simulink model "Potenciometro"  (R2022b)
settings: Solver=VariableStepAuto  StartTime=0.0  StopTime=10.0  RelTol=1e-3
libraries: fl_lib x6, nesl_utility x2, ee_lib x1
settings Model: Creator=matheusassis  LastModifiedBy=matheusassis

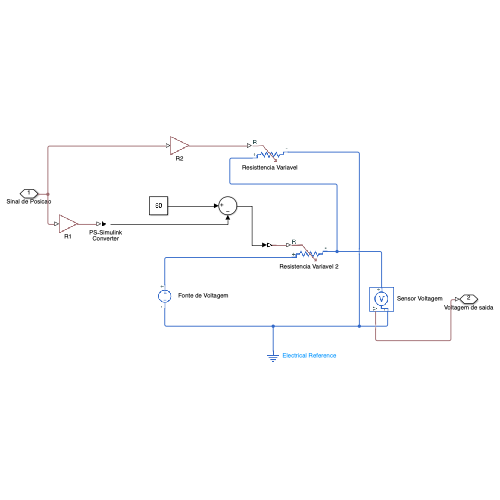
[thumbnail: Simulink's stored preview of the top-level diagram]
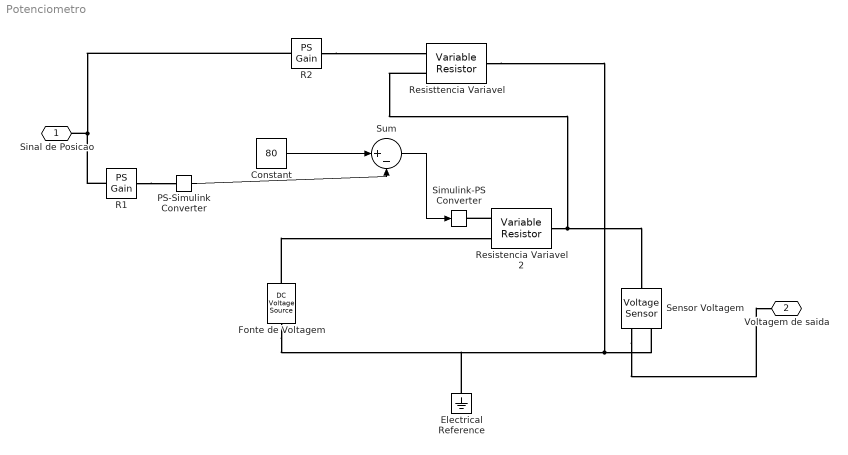
== system Potenciometro ==
  " Fonte de Voltagem" : ee_lib/Additional Components/SPICE Sources/DC Voltage Source  DC=10 V
  Constant : Constant  Value=80
  Electrical Reference : fl_lib/Electrical/Electrical Elements/Electrical Reference
  PS-Simulink Converter : nesl_utility/PS-Simulink Converter  PhysicalDomain=network_engine_domain  SubClassName=ps_output  LeftPortType=input  RightPortType=output  PseudoPeriodic=off  Frequencies=[]  VectorFormat=inherit  Unit=inherit  AffineConversion=off
  R1 : fl_lib/Physical Signals/Functions/PS Gain  gain=1
  R2 : fl_lib/Physical Signals/Functions/PS Gain  gain=1
  Resistencia Variavel 2 : fl_lib/Electrical/Electrical Elements/Variable Resistor  Rmin=0 Ohm  i_specify=off  i_priority=None  i=0 A  i_nominal_specify=off  i_nominal_unit=A  i_nominal_value=1  v_specify=off  v_priority=None  v=0 V  v_nominal_specify=off  v_nominal_unit=V  v_nominal_value=1
  Resisttencia Variavel : fl_lib/Electrical/Electrical Elements/Variable Resistor  Rmin=0 Ohm  i_specify=off  i_priority=None  i=0 A  i_nominal_specify=off  i_nominal_unit=A  i_nominal_value=1  v_specify=off  v_priority=None  v=0 V  v_nominal_specify=off  v_nominal_unit=V  v_nominal_value=1
  "Sensor Voltagem " : fl_lib/Electrical/Electrical Sensors/Voltage Sensor
  Simulink-PS Converter : nesl_utility/Simulink-PS Converter  PhysicalDomain=network_engine_domain  SubClassName=ps_input  LeftPortType=input  RightPortType=output  PseudoPeriodic=off  Frequencies=[]  NoiseDistribution=none  NoiseParameters=[]  Unit=1  AffineConversion=off  FilteringAndDerivatives=provide  SimscapeFilterOrder=1  InputFilterTimeConstant=0.001  UdotUserProvided=0
  Sum : Sum  Inputs=|+-
  Sinal de Posicao : PMIOPort  Side=Left
  Voltagem de saida : PMIOPort  Port=2  Side=Left
  wires:
  PS-Simulink Converter/1 -> Sum/2
  Sum/1 -> Simulink-PS Converter/1
  Constant/1 -> Sum/1
  connections:
  R1/RConn1 -- PS-Simulink Converter/LConn1
  R1/LConn1 -- R2/LConn1 -- Sinal de Posicao/RConn1
  R2/RConn1 -- Resisttencia Variavel/LConn1
  Resistencia Variavel 2/LConn1 -- Simulink-PS Converter/RConn1
  Resisttencia Variavel/RConn1 -- Electrical Reference/LConn1 -- " Fonte de Voltagem"/RConn1 -- "Sensor Voltagem "/RConn2
  Resistencia Variavel 2/RConn1 -- "Sensor Voltagem "/LConn1 -- Resisttencia Variavel/LConn2
  " Fonte de Voltagem"/LConn1 -- Resistencia Variavel 2/LConn2
  "Sensor Voltagem "/RConn1 -- Voltagem de saida/RConn1
